simulink model "SEPIC"  (R2015a)
settings: Solver=ode45  StartTime=0.0  StopTime=10.0  RelTol=1e-3
values from neighbouring files (symbols this model uses):
  C1 = 120e-6    (= 0.00012)    [SEPIC_code.m]
  C2 = 120e-6    (= 0.00012)    [SEPIC_code.m]
  D = 0.5    [SEPIC_code.m]
  L1 = 470e-6    (= 0.00047)    [SEPIC_code.m]
  L2 = 470e-6    (= 0.00047)    [SEPIC_code.m]
  R = 100    [SEPIC_code.m]
  Vd = 12    [SEPIC_code.m]
libraries: powerlib x10, powerlib_meascontrol x1
settings Model: Creator=Daymee  LastModifiedBy=Daymee

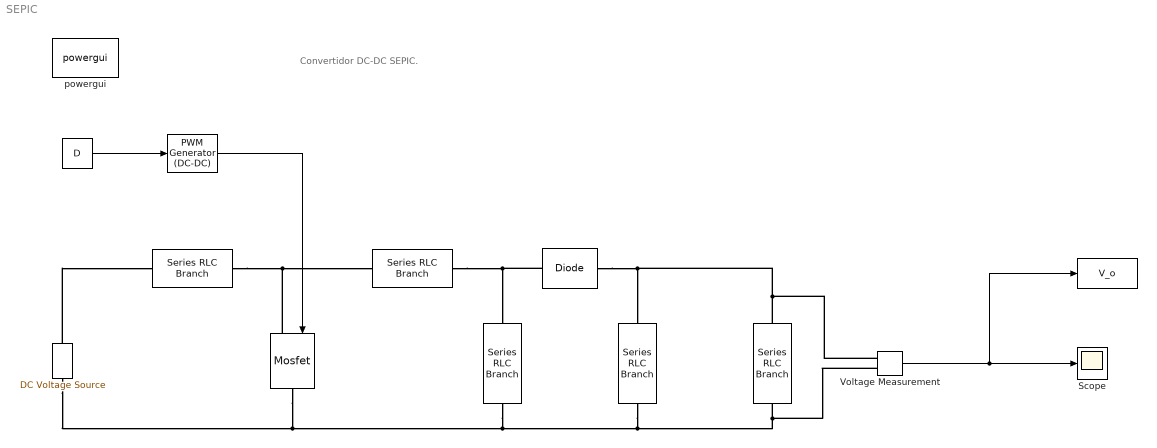
== system SEPIC ==
  note: Convertidor DC-DC SEPIC.
  " " : Constant  Value=D
  "  " : powerlib_meascontrol/Pulse & Signal Generators/PWM Generator (DC-DC)  Fsw=Fs  Ts=0
  "   " : powerlib/Electrical Sources/DC Voltage Source  Amplitude=Vd  Measurements=None
  "    " : powerlib/Elements/Series RLC Branch  LConnTagsString=__new0  RConnTagsString=__new0  BranchType=L  Resistance=1  Inductance=L1  SetiL0=off  InitialCurrent=0  Capacitance=1e-6  Setx0=off  InitialVoltage=0  Measurements=None
  "     " : powerlib/Power Electronics/Mosfet  Ron=0.1  Lon=0  Rd=0.01  Vfd=0  IC=0  Rs=1e5  Cs=inf  Measurements=off
  "      " : powerlib/Elements/Series RLC Branch  LConnTagsString=__new0  RConnTagsString=__new0  BranchType=L  Resistance=1  Inductance=L2  SetiL0=off  InitialCurrent=0  Capacitance=1e-6  Setx0=off  InitialVoltage=0  Measurements=None
  "        " : powerlib/Elements/Series RLC Branch  LConnTagsString=__new0  RConnTagsString=__new0  BranchType=C  Resistance=1  Inductance=1e-3  SetiL0=off  InitialCurrent=0  Capacitance=C1  Setx0=off  InitialVoltage=0  Measurements=None
  "          " : powerlib/Elements/Series RLC Branch  LConnTagsString=__new0  RConnTagsString=__new0  BranchType=C  Resistance=1  Inductance=1e-3  SetiL0=off  InitialCurrent=0  Capacitance=C2  Setx0=off  InitialVoltage=0  Measurements=None
  "             " : powerlib/Elements/Series RLC Branch  LConnTagsString=__new0  RConnTagsString=__new0  BranchType=R  Resistance=R  Inductance=1e-3  SetiL0=off  InitialCurrent=0  Capacitance=1e-6  Setx0=off  InitialVoltage=0  Measurements=None
  "                                       " : ToWorkspace  VariableName=V_o  SampleTime=-1
  "                                           " : powerlib/Power Electronics/Diode  Ron=0.001  Lon=0  Vf=0.8  IC=0  UseSnubber=off  Rs=500  Cs=250e-9  Measurements=off
  Scope : Scope
  Voltage Measurement : powerlib/Measurements/Voltage Measurement  PhasorSimulation=off  OutputType=Complex  PSBequivalent=0
  powergui : powerlib/powergui  Priority=1  SimulationMode=Continuous  SolverType=Tustin/Backward Euler (TBE)  SampleTime=50e-6  frequency=60  SPID=off  DisableSnubberDevices=off  DisableRonSwitches=off  DisableVfSwitches=off  SwTol=0  DisplayEquations=off  Interpol=off  methode=off  Ts=100  FunctionMessages=off  echomessages=off  HookPort=off  EnableUseOfTLC=off  x0status=blocks  frequencyindice=60  Pbase=100e6  ErrMax=1e-4  Iterations=50  UnitsV=kV  UnitsW=MW  buscounter=0  RestoreLinks=warning  ResistiveCurrentMeasurement=off  Frange=[0:2:500]  Ylog=off  Xlog=on  ShowGrid=off  save=off  variable=ZData  structure=0  ZoomFFT=off  StartTime=0.0  cycles=1  DisplayStyle=1  fundamental=60  FreqAxis=off  MaxFrequency=1000  frequencyindicesteady=1  RmsSteady=1  display=off
  wires:
  "  "/1 -> "     "/1
  " "/1 -> "  "/1
  Voltage Measurement/1 -> "                                       "/1, Scope/1
  connections:
  "   "/RConn1 -- "    "/LConn1
  "    "/RConn1 -- "     "/LConn1 -- "        "/LConn1
  "        "/RConn1 -- "                                           "/LConn1 -- "      "/LConn1
  "   "/LConn1 -- "     "/RConn1 -- "      "/RConn1 -- "          "/RConn1 -- Voltage Measurement/LConn2 -- "             "/RConn1
  "             "/LConn1 -- Voltage Measurement/LConn1 -- "                                           "/RConn1 -- "          "/LConn1
